simulink model "Inversor_full_bridge_2"  (R2015a)
settings: Solver=ode23tb  StartTime=0.0  StopTime=0.01  MaxStep=0.5e-5  RelTol=1e-3
libraries: powerlib x11, simulink x1
settings Model: Creator=Leandro  LastModifiedBy=Iury
settings DataIOCC: SignalLoggingSaveFormat=ModelDataLogs
settings DebuggingCC: UnderspecifiedInitializationDetection=Classic  MergeDetectMultiDrivingBlocksExec=none  SolverPrmCheckMsg=warning  FcnCallInpInsideContextMsg=UseLocalSettings  StateNameClashWarn=warning
settings SFSimCC: SimCustomHeaderCode="#include \"controle.h\""  SimUserSources=controle.c
settings GRTTargetCC: CombineOutputUpdateFcns=off  GRTInterface=on

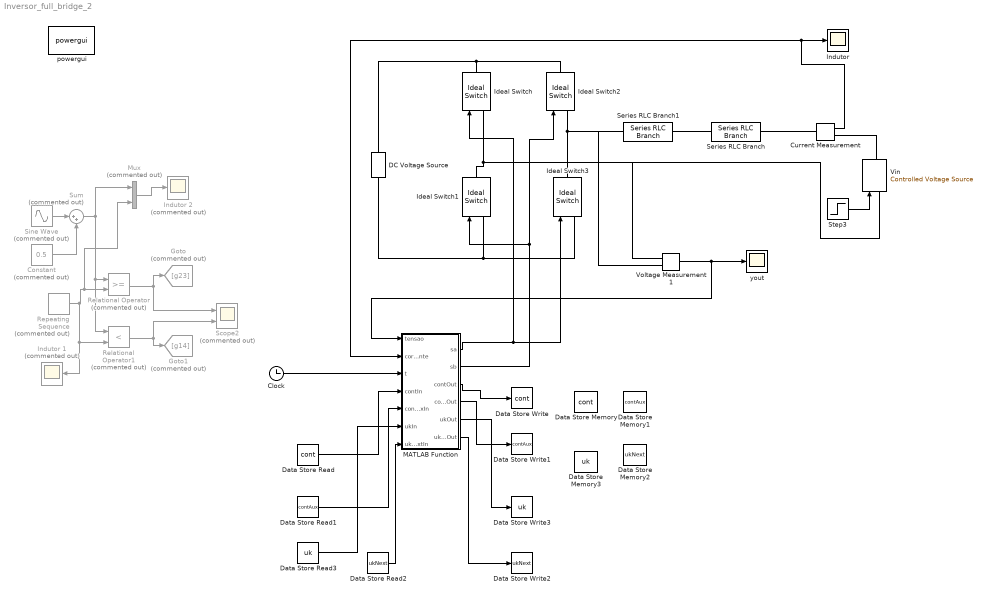
== system Inversor_full_bridge_2 ==
  Clock : Clock
  Constant : Constant  Commented=on  Value=0.5
  Current Measurement : powerlib/Measurements/Current Measurement  PhasorSimulation=off  OutputType=Complex  PSBequivalent=0
  DC Voltage Source : powerlib/Electrical Sources/DC Voltage Source  Amplitude=200  Measurements=None
  Data Store Memory : DataStoreMemory  DataStoreName=cont  ReadBeforeWriteMsg=warning  WriteAfterWriteMsg=warning  WriteAfterReadMsg=warning  InitialValue=1
  Data Store Memory1 : DataStoreMemory  DataStoreName=contAux  ReadBeforeWriteMsg=warning  WriteAfterWriteMsg=warning  WriteAfterReadMsg=warning  InitialValue=1
  Data Store Memory2 : DataStoreMemory  DataStoreName=ukNext  ReadBeforeWriteMsg=warning  WriteAfterWriteMsg=warning  WriteAfterReadMsg=warning
  Data Store Memory3 : DataStoreMemory  DataStoreName=uk  ReadBeforeWriteMsg=warning  WriteAfterWriteMsg=warning  WriteAfterReadMsg=warning
  Data Store Read : DataStoreRead  DataStoreName=cont
  Data Store Read1 : DataStoreRead  DataStoreName=contAux
  Data Store Read2 : DataStoreRead  DataStoreName=ukNext
  Data Store Read3 : DataStoreRead  DataStoreName=uk
  Data Store Write : DataStoreWrite  DataStoreName=cont
  Data Store Write1 : DataStoreWrite  DataStoreName=contAux
  Data Store Write2 : DataStoreWrite  DataStoreName=ukNext
  Data Store Write3 : DataStoreWrite  DataStoreName=uk
  Goto : Goto  Commented=on  GotoTag=g23
  Goto1 : Goto  Commented=on  GotoTag=g14
  Ideal Switch{,1..3} (4 alike) : powerlib/Power Electronics/Ideal Switch  Ron=1e-6  Lon=0  IC=0  Rs=1e5  Cs=inf  Measurements=off
  "Indutor " : Scope
      settings: TimeRange=0.01  YMin=-671  YMax=-664.5  SaveName=i
  Indutor 1 : Scope  Commented=on
      settings: TimeRange=0.05  YMin=0  YMax=20  SaveName=i1
  Indutor 2 : Scope  Commented=on
      settings: TimeRange=0.05  YMin=0  YMax=20  SaveName=i2
  MATLAB Function : MATLAB Function  TreatAsAtomicUnit=on
  Mux : Mux  Commented=on  Inputs=2
  Relational Operator : RelationalOperator  Commented=on  OutDataTypeStr=boolean
  Relational Operator1 : RelationalOperator  Commented=on  Operator=<  OutDataTypeStr=boolean
  Repeating Sequence : simulink/Sources/Repeating Sequence  Commented=on  rep_seq_t=[0 1/20000 1/10000]  rep_seq_y=[0 1 0]
  Scope2 : Scope  Commented=on  NumInputPorts=2
      settings: TimeRange=0.05  YMin=0~0  YMax=1~1  SaveName=ScopeData2
  Series RLC Branch : powerlib/Elements/Series RLC Branch  LConnTagsString=__new0  RConnTagsString=__new0  BranchType=L  Resistance=0  Inductance=2e-3  SetiL0=off  InitialCurrent=0  Capacitance=1.0  Setx0=off  InitialVoltage=0  Measurements=None
  Series RLC Branch1 : powerlib/Elements/Series RLC Branch  LConnTagsString=__new0  RConnTagsString=__new0  BranchType=R  Resistance=0.1  Inductance=2e-3  SetiL0=off  InitialCurrent=0  Capacitance=1.0  Setx0=off  InitialVoltage=0  Measurements=None
  Sine Wave : Sin  Commented=on  Amplitude=0.3  Frequency=60*2*pi  SampleTime=0
  Step3 : Step  Time=0  After=0  SampleTime=0
  Sum : Sum  Commented=on  Inputs=|++
  Vin : powerlib/Electrical Sources/Controlled Voltage Source  Initialize=on  Source_Type=AC  Amplitude=0  Phase=0  Frequency=0  Measurements=None
  Voltage Measurement1 : powerlib/Measurements/Voltage Measurement  PhasorSimulation=off  OutputType=Complex  PSBequivalent=0
  powergui : powerlib/powergui  Priority=1  SimulationMode=Continuous  SolverType=Tustin  SampleTime=50e-6  frequency=60  SPID=on  DisableSnubberDevices=off  DisableRonSwitches=off  DisableVfSwitches=off  SwTol=0  DisplayEquations=off  Interpol=off  methode=off  Ts=0  FunctionMessages=off  echomessages=off  HookPort=off  EnableUseOfTLC=off  x0status=blocks  frequencyindice=0  Pbase=100e6  ErrMax=1e-4  Iterations=50  UnitsV=kV  UnitsW=MW  buscounter=0  RestoreLinks=warning  ResistiveCurrentMeasurement=off  Frange=[0:2:500]  Ylog=off  Xlog=on  ShowGrid=off  save=off  variable=ZData  structure=0  ZoomFFT=off  StartTime=0.0  cycles=1  DisplayStyle=1  fundamental=60  FreqAxis=off  MaxFrequency=1000  frequencyindicesteady=1  RmsSteady=1  display=off
  yout : Scope
      settings: YMin=199.999  YMax=199.999
  wires:
  MATLAB Function/2(sb) -> Ideal Switch2/1, Ideal Switch1/1
  MATLAB Function/1(sa) -> Ideal Switch3/1, Ideal Switch/1
  Current Measurement/1 -> MATLAB Function/2(corrente), "Indutor "/1
  Voltage Measurement1/1 -> yout/1, MATLAB Function/1(tensao)
  Step3/1 -> Vin/1
  Clock/1 -> MATLAB Function/3(t)
  Data Store Read/1 -> MATLAB Function/4(contIn)
  MATLAB Function/3(contOut) -> Data Store Write/1
  MATLAB Function/4(contAuxOut) -> Data Store Write1/1
  Data Store Read1/1 -> MATLAB Function/5(contAuxIn)
  Data Store Read3/1 -> MATLAB Function/6(ukIn)
  Data Store Read2/1 -> MATLAB Function/7(ukNextIn)
  MATLAB Function/6(ukNextOut) -> Data Store Write2/1
  MATLAB Function/5(ukOut) -> Data Store Write3/1
  Repeating Sequence/1 -> Indutor 1/1, Relational Operator1/2, Mux/2, Relational Operator/2
  Relational Operator/1 -> Goto/1, Scope2/1
  Relational Operator1/1 -> Goto1/1, Scope2/2
  Sine Wave/1 -> Sum/1
  Constant/1 -> Sum/2
  Sum/1 -> Relational Operator1/1, Relational Operator/1, Mux/1
  Mux/1 -> Indutor 2/1
  connections:
  Series RLC Branch/RConn1 -- Current Measurement/LConn1
  Ideal Switch3/RConn1 -- Voltage Measurement1/LConn2 -- Series RLC Branch1/RConn1 -- Ideal Switch2/LConn1
  Ideal Switch2/RConn1 -- DC Voltage Source/RConn1 -- Ideal Switch/RConn1
  Ideal Switch3/LConn1 -- DC Voltage Source/LConn1 -- Ideal Switch1/LConn1
  Ideal Switch1/RConn1 -- Voltage Measurement1/LConn1 -- Vin/LConn1 -- Ideal Switch/LConn1
  Series RLC Branch1/LConn1 -- Series RLC Branch/LConn1
  Current Measurement/RConn1 -- Vin/RConn1

== matlab function Inversor_full_bridge_2/MATLAB Function ==
  data: tensao input; sa output; sb output; corrente input; t input; contIn input; contOut output; contAuxIn input; contAuxOut output; ukOut output; ukIn input; ukNextIn input; ukNextOut output
function [sa,sb,contOut, contAuxOut, ukOut, ukNextOut]= fcn(tensao, corrente, t, contIn, contAuxIn,ukIn, ukNextIn)

k1 = -22.626994881450905;
k2 = -0.561421978901323;
k3 = 79.163345802203452;
k4 = -76.791082664183065;

persistent pontosig;
pontosig = 167;

pi = 3.14159265;
Sd11 = 0.03125;
Sd21 = 0;
Rd11 = 1.998579261776922;
Rd21 = 1;
Rd12 = -0.999999980007103;
Rd22 = 0;

% Variáveis
t_ks = 0;	                  		
n = 0;
pontos_am = 0;
modul_ma_k = 0;
modul_ma_nxt1 = 0;
v_abf_k = 0;
ig_k = 0;
ig_ref_ks=0;
ig_ref_k=0;
Vcc = 200;
ig_ref_nxt2 = 0;
ig_cont_nxt1 = 0;
ig_ref_amost_ks = 0;
v_tri = 0;
sa = 0;
sb = 0;
u_ks=0;
x_ks=0;
theta_ks=0;
rho1_ks=0;
rho2_ks=0;
Rf = 0.1;
Lf = 0.005;
Ig_pk = 10;
theta = 0;
w = 376.99;
u_k=0.5;
u_nxt1=0.5;
cont = contIn;
cont_aux = contAuxIn;

persistent TPER;

rho1_ks_nxt=0;
rho2_ks_nxt=0;
Fs = 10000;
Ts = 1.0e-4;		
Fsw = 10000;
Tsw = 1.0e-4;      
Pontos_fs = 200;  
Pontos_fsw = 200;
persistent t_sample;
t_sample = 200;

ig_ref_k = Ig_pk*sin(w*t);
     
%Controlador
if t_sample == Pontos_fs 
	ig_k = corrente;
	v_abf_k = tensao;
		
	rho1_ks = rho1_ks_nxt;
	rho2_ks = rho2_ks_nxt;
		
    ig_ref_ks = ig_ref_k;
        
    modul_ma_k = modul_ma_nxt1;
    
   % u_k = u_nxt1;
   
       
   % modul_ma_nxt1 = k1*ig_k + k2*modul_ma_k + k3*rho1_ks + k4*rho2_ks;
    %u_nxt1 = (modul_ma_nxt1/(2*Vcc))+0.5;
  
        
   % rho1_ks_nxt = -Sd11*ig_k + 0*modul_ma_k + Rd11*rho1_ks + Rd12*rho2_ks + 0*modul_ma_nxt1 + Sd11 * ig_ref_ks;
    %rho2_ks_nxt = -Sd21*ig_k + 0*modul_ma_k + Rd21*rho1_ks + Rd22*rho2_ks + 0*modul_ma_nxt1 + Sd21 * ig_ref_ks;
        
    x_ks = ig_k;
    t_ks = t_ks + Ts;   
    
end

 %Modulador DSP

    TPER = Pontos_fsw/2;   % PWM simétrico (triangular)
       
    if cont_aux < Pontos_fsw
       cont_aux=cont_aux+1;
    else
       cont_aux=1; 
    end
          
    if cont_aux < TPER
       cont = cont+1;
    elseif cont_aux >= TPER && cont_aux < Pontos_fsw
         cont = cont-1;
    else 
       cont=1;
    end
      
    if u_k*TPER >= cont
       sa=1;
    else
       sa=0;
    end
       
    sb=1-sa;

    
    contOut = cont;
    contAuxOut = cont_aux;
    ukOut = u_k;
    ukNextOut = u_nxt1;
    
    t_sample = t_sample + 1;
end
